simulink model "fordbfs"  (R2021b)
settings: Solver=VariableStepAuto  StartTime=0.0  RelTol=1e-3
libraries: dspfdesign x12, dspmathops x12, dspvision x2, dspsnks4 x1
settings Model: PacingRate=100  Creator=DSP  LastModifiedBy=teyji

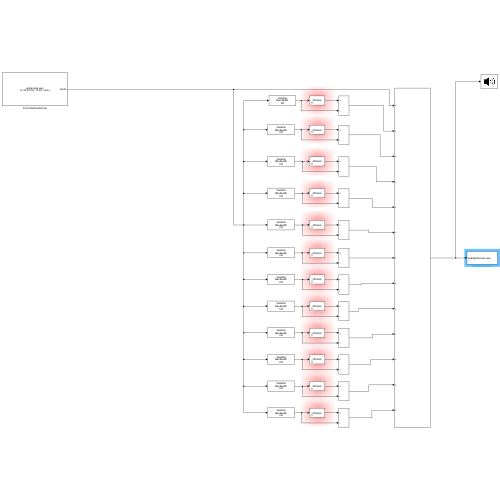
[thumbnail: Simulink's stored preview of the top-level diagram]
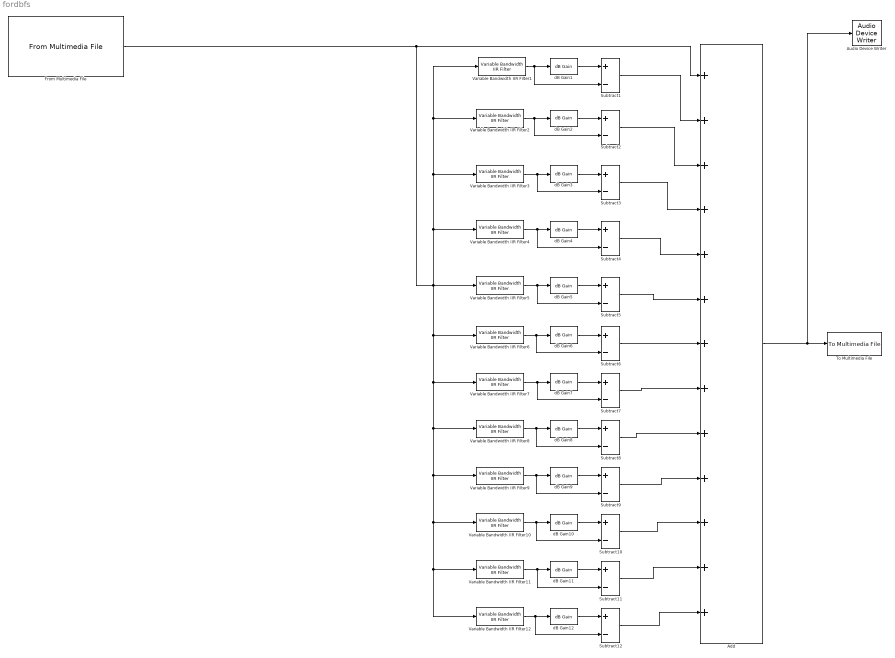
== system fordbfs ==
  Add : Sum  Inputs=+++++++++++++
  Audio Device Writer : dspsnks4/Audio Device Writer  Driver=DirectSound  Device=Default  InheritSampleRate=on  SampleRate=44100  BitDepth=16-bit integer  BufferSize=4096  NumBuffers=10  DefaultOutputChannelMapping=on  OutputChannelMapping=1:2  OutputNumUnderrunSamples=off  DriverIdx=1  DeviceWarnFlag=''
  From Multimedia File : dspvision/From Multimedia File  inputFilename=whitenoise.wav  readRange=[1 Inf]  loop=on  numPlays=inf  outputStreams=Audio only  videoDataType=single  audioDataType=double  inheritSampleTime=on  userDefinedSampleTime=1/30  noAudioOutput=off  isIntensityVideo=off  fourcc=RGB  colorVideoFormat=Separate color signals  outputEOF=off  dataOrg=Column-major  audioFrameSize=1024  computeAudioFrameSize=off  outSamplingMode=Sample based
  Subtract{1..12} (12 alike) : Sum  Inputs=+-
  To Multimedia File : dspvision/To Multimedia File  outputFilename=�whitenoise.wav  streamSelection=Audio only  videoCompressor=None (uncompressed)  audioCompressor=None (uncompressed)  imagePorts=Separate color signals  fileType=WAV  audioDatatype=16-bit integer  fourcc=RGB  videoQuality=75  mj2000CompFactor=10
  Variable Bandwidth IIR Filter1 : dspfdesign/Variable Bandwidth IIR Filter  FilterType=Bandpass  FilterOrder=4  PassbandFrequencyPort=off  PassbandFrequency=512  CenterFrequencyPort=off  CenterFrequency=100  BandwidthPort=off  Bandwidth=10  PassbandRipple=1  StopbandAttenuation=60  InheritSampleRate=off  SampleRate=44100  SimulateUsing=Code generation
      settings: SourceProductBaseCode=DS
  Variable Bandwidth IIR Filter10 : dspfdesign/Variable Bandwidth IIR Filter  FilterType=Bandpass  FilterOrder=4  PassbandFrequencyPort=off  PassbandFrequency=512  CenterFrequencyPort=off  CenterFrequency=800  BandwidthPort=off  Bandwidth=91  PassbandRipple=1  StopbandAttenuation=60  InheritSampleRate=off  SampleRate=44100  SimulateUsing=Code generation
      settings: SourceProductBaseCode=DS
  Variable Bandwidth IIR Filter11 : dspfdesign/Variable Bandwidth IIR Filter  FilterType=Bandpass  FilterOrder=4  PassbandFrequencyPort=off  PassbandFrequency=512  CenterFrequencyPort=off  CenterFrequency=1000  BandwidthPort=off  Bandwidth=110  PassbandRipple=1  StopbandAttenuation=60  InheritSampleRate=off  SampleRate=44100  SimulateUsing=Code generation
      settings: SourceProductBaseCode=DS
  Variable Bandwidth IIR Filter12 : dspfdesign/Variable Bandwidth IIR Filter  FilterType=Bandpass  FilterOrder=4  PassbandFrequencyPort=off  PassbandFrequency=512  CenterFrequencyPort=off  CenterFrequency=1250  BandwidthPort=off  Bandwidth=130  PassbandRipple=1  StopbandAttenuation=60  InheritSampleRate=off  SampleRate=44100  SimulateUsing=Code generation
      settings: SourceProductBaseCode=DS
  Variable Bandwidth IIR Filter2 : dspfdesign/Variable Bandwidth IIR Filter  FilterType=Bandpass  FilterOrder=4  PassbandFrequencyPort=off  PassbandFrequency=512  CenterFrequencyPort=off  CenterFrequency=125  BandwidthPort=off  Bandwidth=15  PassbandRipple=1  StopbandAttenuation=60  InheritSampleRate=off  SampleRate=44100  SimulateUsing=Code generation
      settings: SourceProductBaseCode=DS
  Variable Bandwidth IIR Filter3 : dspfdesign/Variable Bandwidth IIR Filter  FilterType=Bandpass  FilterOrder=4  PassbandFrequencyPort=off  PassbandFrequency=512  CenterFrequencyPort=off  CenterFrequency=160  BandwidthPort=off  Bandwidth=18  PassbandRipple=1  StopbandAttenuation=60  InheritSampleRate=off  SampleRate=44100  SimulateUsing=Code generation
      settings: SourceProductBaseCode=DS
  Variable Bandwidth IIR Filter4 : dspfdesign/Variable Bandwidth IIR Filter  FilterType=Bandpass  FilterOrder=4  PassbandFrequencyPort=off  PassbandFrequency=512  CenterFrequencyPort=off  CenterFrequency=200  BandwidthPort=off  Bandwidth=25  PassbandRipple=1  StopbandAttenuation=60  InheritSampleRate=off  SampleRate=44100  SimulateUsing=Code generation
      settings: SourceProductBaseCode=DS
  Variable Bandwidth IIR Filter5 : dspfdesign/Variable Bandwidth IIR Filter  FilterType=Bandpass  FilterOrder=4  PassbandFrequencyPort=off  PassbandFrequency=512  CenterFrequencyPort=off  CenterFrequency=250  BandwidthPort=off  Bandwidth=30  PassbandRipple=1  StopbandAttenuation=60  InheritSampleRate=off  SampleRate=44100  SimulateUsing=Code generation
      settings: SourceProductBaseCode=DS
  Variable Bandwidth IIR Filter6 : dspfdesign/Variable Bandwidth IIR Filter  FilterType=Bandpass  FilterOrder=4  PassbandFrequencyPort=off  PassbandFrequency=512  CenterFrequencyPort=off  CenterFrequency=315  BandwidthPort=off  Bandwidth=38  PassbandRipple=1  StopbandAttenuation=60  InheritSampleRate=off  SampleRate=44100  SimulateUsing=Code generation
      settings: SourceProductBaseCode=DS
  Variable Bandwidth IIR Filter7 : dspfdesign/Variable Bandwidth IIR Filter  FilterType=Bandpass  FilterOrder=4  PassbandFrequencyPort=off  PassbandFrequency=512  CenterFrequencyPort=off  CenterFrequency=400  BandwidthPort=off  Bandwidth=45  PassbandRipple=1  StopbandAttenuation=60  InheritSampleRate=off  SampleRate=44100  SimulateUsing=Code generation
      settings: SourceProductBaseCode=DS
  Variable Bandwidth IIR Filter8 : dspfdesign/Variable Bandwidth IIR Filter  FilterType=Bandpass  FilterOrder=4  PassbandFrequencyPort=off  PassbandFrequency=512  CenterFrequencyPort=off  CenterFrequency=500  BandwidthPort=off  Bandwidth=60  PassbandRipple=1  StopbandAttenuation=60  InheritSampleRate=off  SampleRate=44100  SimulateUsing=Code generation
      settings: SourceProductBaseCode=DS
  Variable Bandwidth IIR Filter9 : dspfdesign/Variable Bandwidth IIR Filter  FilterType=Bandpass  FilterOrder=4  PassbandFrequencyPort=off  PassbandFrequency=512  CenterFrequencyPort=off  CenterFrequency=630  BandwidthPort=off  Bandwidth=72  PassbandRipple=1  StopbandAttenuation=60  InheritSampleRate=off  SampleRate=44100  SimulateUsing=Code generation
      settings: SourceProductBaseCode=DS
  dB Gain1 : dspmathops/dB Gain  dB=gain1  intype=Amplitude
      settings: SourceProductBaseCode=DS
  dB Gain10 : dspmathops/dB Gain  dB=gain10  intype=Amplitude
      settings: SourceProductBaseCode=DS
  dB Gain11 : dspmathops/dB Gain  dB=gain11  intype=Amplitude
      settings: SourceProductBaseCode=DS
  dB Gain12 : dspmathops/dB Gain  dB=gain12  intype=Amplitude
      settings: SourceProductBaseCode=DS
  dB Gain2 : dspmathops/dB Gain  dB=gain2  intype=Amplitude
      settings: SourceProductBaseCode=DS
  dB Gain3 : dspmathops/dB Gain  dB=gain3  intype=Amplitude
      settings: SourceProductBaseCode=DS
  dB Gain4 : dspmathops/dB Gain  dB=gain4  intype=Amplitude
      settings: SourceProductBaseCode=DS
  dB Gain5 : dspmathops/dB Gain  dB=gain5  intype=Amplitude
      settings: SourceProductBaseCode=DS
  dB Gain6 : dspmathops/dB Gain  dB=gain6  intype=Amplitude
      settings: SourceProductBaseCode=DS
  dB Gain7 : dspmathops/dB Gain  dB=gain7  intype=Amplitude
      settings: SourceProductBaseCode=DS
  dB Gain8 : dspmathops/dB Gain  dB=gain8  intype=Amplitude
      settings: SourceProductBaseCode=DS
  dB Gain9 : dspmathops/dB Gain  dB=gain9  intype=Amplitude
      settings: SourceProductBaseCode=DS
  wires:
  Variable Bandwidth IIR Filter1/1 -> Subtract1/2, dB Gain1/1
  Variable Bandwidth IIR Filter2/1 -> Subtract2/2, dB Gain2/1
  Variable Bandwidth IIR Filter3/1 -> Subtract3/2, dB Gain3/1
  dB Gain1/1 -> Subtract1/1
  Subtract1/1 -> Add/2
  dB Gain2/1 -> Subtract2/1
  dB Gain3/1 -> Subtract3/1
  Subtract2/1 -> Add/3
  Subtract3/1 -> Add/4
  Variable Bandwidth IIR Filter4/1 -> Subtract4/2, dB Gain4/1
  Variable Bandwidth IIR Filter5/1 -> Subtract5/2, dB Gain5/1
  dB Gain4/1 -> Subtract4/1
  dB Gain5/1 -> Subtract5/1
  Subtract4/1 -> Add/5
  Subtract5/1 -> Add/6
  Variable Bandwidth IIR Filter6/1 -> Subtract6/2, dB Gain6/1
  Variable Bandwidth IIR Filter7/1 -> Subtract7/2, dB Gain7/1
  Variable Bandwidth IIR Filter8/1 -> Subtract8/2, dB Gain8/1
  dB Gain6/1 -> Subtract6/1
  dB Gain7/1 -> Subtract7/1
  dB Gain8/1 -> Subtract8/1
  dB Gain9/1 -> Subtract9/1
  Variable Bandwidth IIR Filter9/1 -> Subtract9/2, dB Gain9/1
  dB Gain10/1 -> Subtract10/1
  Variable Bandwidth IIR Filter10/1 -> Subtract10/2, dB Gain10/1
  dB Gain11/1 -> Subtract11/1
  Variable Bandwidth IIR Filter11/1 -> Subtract11/2, dB Gain11/1
  Variable Bandwidth IIR Filter12/1 -> Subtract12/2, dB Gain12/1
  dB Gain12/1 -> Subtract12/1
  Subtract6/1 -> Add/7
  Subtract7/1 -> Add/8
  Subtract8/1 -> Add/9
  Subtract9/1 -> Add/10
  Subtract10/1 -> Add/11
  Subtract11/1 -> Add/12
  Subtract12/1 -> Add/13
  From Multimedia File/1 -> Add/1, Variable Bandwidth IIR Filter1/1, Variable Bandwidth IIR Filter2/1, Variable Bandwidth IIR Filter3/1, Variable Bandwidth IIR Filter4/1, Variable Bandwidth IIR Filter12/1, Variable Bandwidth IIR Filter11/1, Variable Bandwidth IIR Filter10/1, Variable Bandwidth IIR Filter9/1, Variable Bandwidth IIR Filter8/1, Variable Bandwidth IIR Filter7/1, Variable Bandwidth IIR Filter6/1, Variable Bandwidth IIR Filter5/1
  Add/1 -> To Multimedia File/1, Audio Device Writer/1
